simulink model "posture_reg"  (Simulink 8.7)
settings: Solver=ode45  StartTime=0.0  StopTime=T  MaxStep=0.01  RelTol=1e-3
values from neighbouring files (symbols this model uses):
  theta_0 = 0    [init.m]
  x_0 = 2    [init.m]
  y_0 = 0    [init.m]
undefined symbols (not defined in the file or in its folder): post_reg, wrap
settings Model: Creator=marilena  LastModifiedBy=giuseppe  ExtModeAutoUpdateStatusClock=off
settings DataIOCC: SignalLoggingSaveFormat=ModelDataLogs
settings OptimizationCC: ExpressionDepthLimit=2147483647
settings DebuggingCC: SaveWithParameterizedLinksMsg=none  SolverPrmCheckMsg=warning  FcnCallInpInsideContextMsg=UseLocalSettings  StateNameClashWarn=warning
settings HardwareCC: TargetHWDeviceType=32-bit Generic
settings GRTTargetCC: TargetFcnLib=ansi_tfl_tmw.mat  GeneratePreprocessorConditionals=Use local settings  CombineOutputUpdateFcns=off  GRTInterface=on

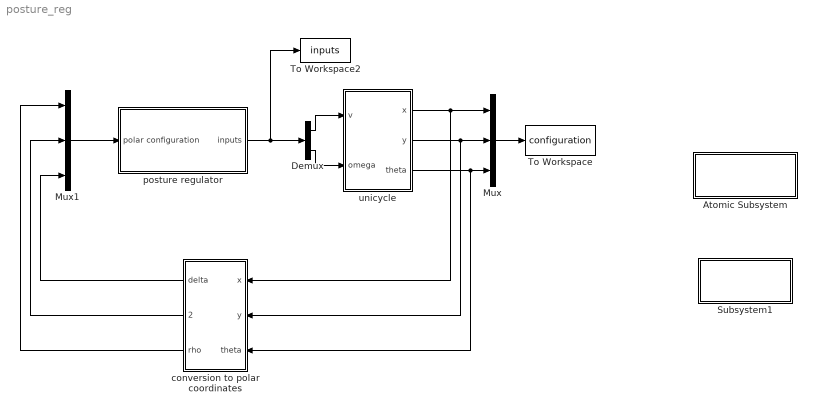
== system posture_reg ==
  Atomic Subsystem : Subsystem  TreatAsAtomicUnit=on
      settings: OpenFcn=init
      mask Display: disp('initialization')
  Demux : Demux  Outputs=2
  Mux : Mux  Inputs=3
  Mux1 : Mux  Inputs=3
  Subsystem1 : Subsystem
      settings: OpenFcn=plots
      mask Display: disp('plots')
  To Workspace : ToWorkspace  VariableName=configuration  SaveFormat=Structure With Time
  To Workspace2 : ToWorkspace  VariableName=inputs  SaveFormat=Structure With Time
  conversion to polar coordinates : Subsystem
  posture regulator : Subsystem
  unicycle : Subsystem
  wires:
  Mux/1 -> To Workspace/1
  Mux1/1 -> posture regulator/1(polar configuration)
  posture regulator/1(inputs) -> Demux/1, To Workspace2/1
  Demux/1 -> unicycle/1(v)
  Demux/2 -> unicycle/2(omega)
  unicycle/1(x) -> conversion to polar coordinates/1(x), Mux/1
  unicycle/2(y) -> conversion to polar coordinates/2(y), Mux/2
  unicycle/3(theta) -> conversion to polar coordinates/3(theta), Mux/3
  conversion to polar coordinates/1(delta) -> Mux1/3
  conversion to polar coordinates/2(gamma) -> Mux1/2
  conversion to polar coordinates/3(rho) -> Mux1/1

== system posture_reg/Atomic Subsystem ==

== system posture_reg/Subsystem1 ==

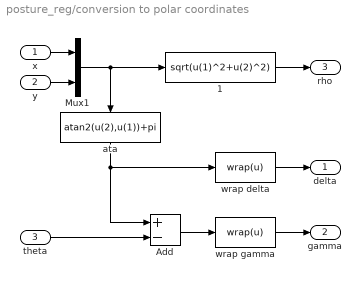
== system posture_reg/conversion to polar coordinates ==
  x : Inport
  y : Inport  Port=2
  theta : Inport  Port=3
  " 1" : Fcn  Expr=sqrt(u(1)^2+u(2)^2)
  Add : Sum  Inputs=+-
  Mux1 : Mux  Inputs=2
  ata : Fcn  Expr=atan2(u(2),u(1))+pi
  wrap delta : MATLABFcn  MATLABFcn=wrap(u)
  wrap gamma : MATLABFcn  MATLABFcn=wrap(u)
  delta : Outport
  gamma : Outport  Port=2
  rho : Outport  Port=3
  wires:
  Mux1/1 -> " 1"/1, ata/1
  ata/1 -> Add/1, wrap delta/1
  x/1 -> Mux1/1
  " 1"/1 -> rho/1
  y/1 -> Mux1/2
  theta/1 -> Add/2
  wrap delta/1 -> delta/1
  Add/1 -> wrap gamma/1
  wrap gamma/1 -> gamma/1

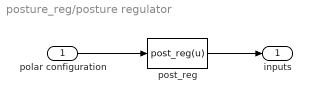
== system posture_reg/posture regulator ==
  polar configuration : Inport
  post_reg : MATLABFcn  Tag={'prova'}  Description=cartesian regulator  MATLABFcn=post_reg(u)  Output1D=off
  inputs : Outport
  wires:
  polar configuration/1 -> post_reg/1
  post_reg/1 -> inputs/1

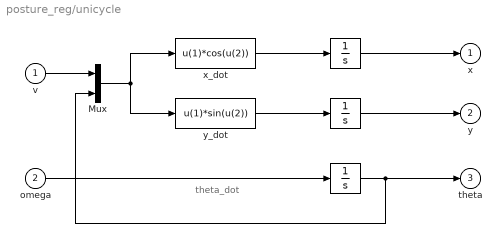
== system posture_reg/unicycle ==
  note: theta_dot
  v : Inport
  omega : Inport  Port=2
  " " : Integrator  InitialCondition=theta_0
  "   " : Integrator  InitialCondition=x_0
  "    " : Integrator  InitialCondition=y_0
  Mux : Mux  Inputs=2
  x_dot : Fcn  Expr=u(1)*cos(u(2))
  y_dot : Fcn  Expr=u(1)*sin(u(2))
  x : Outport
  y : Outport  Port=2
  theta : Outport  Port=3
  wires:
  v/1 -> Mux/1
  omega/1 -> " "/1
  x_dot/1 -> "   "/1
  y_dot/1 -> "    "/1
  " "/1 -> Mux/2, theta/1
  Mux/1 -> x_dot/1, y_dot/1
  "   "/1 -> x/1
  "    "/1 -> y/1
